simulink model "Loisaga_DAM_Simulink_No6"  (R2023b)
settings: Solver=VariableStepAuto  StartTime=0.0  StopTime=20  RelTol=1e-3
values from neighbouring files (symbols this model uses):
  G_DEN6 = [1 2 3 4 1]    [Loisaga_DAM_MatLab_No3and6.m]
  G_NUM6 = [4 3 2 1]    [Loisaga_DAM_MatLab_No3and6.m]
settings Model: Creator=Mark Bejasa  LastModifiedBy=Mark Bejasa

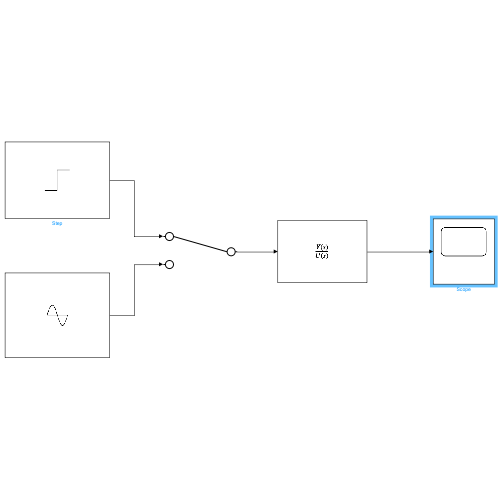
[thumbnail: Simulink's stored preview of the top-level diagram]
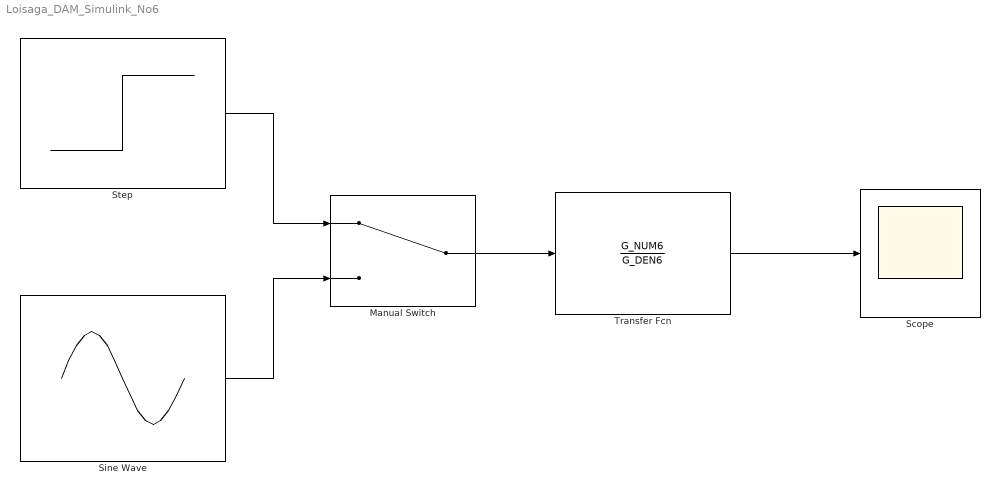
== system Loisaga_DAM_Simulink_No6 ==
  Manual Switch : ManualSwitch
  Scope : Scope
  Sine Wave : Sin  SampleTime=0
  Step : Step  SampleTime=0
  Transfer Fcn : TransferFcn  Numerator=G_NUM6  Denominator=G_DEN6
  wires:
  Step/1 -> Manual Switch/1
  Sine Wave/1 -> Manual Switch/2
  Manual Switch/1 -> Transfer Fcn/1
  Transfer Fcn/1 -> Scope/1
